simulink model "valid_rst"  (Simulink 9.2)
settings: Solver=ode45  StartTime=0.0  StopTime=1.0  RelTol=1e-3  EnableMultiTasking=on
values from neighbouring files (symbols this model uses):
  Ks = 0.157    [nxt_rst.m]
  R = double(vpa(coeffs(collect(expand(eval(Ax*R0))),z_),Acc))    [nxt_rst.m]
  S = double(vpa(coeffs(collect(expand(eval((1-z_)^p*Bx*S2))),z_),Acc))    [nxt_rst.m]
  T = double(vpa(coeffs(collect(expand(eval(Ax*T0))),z_),Acc))    [nxt_rst.m]
  tau = 0.0667    [nxt_rst.m]
  Te = 0.01    [nxt_rst.m]
settings Model: Creator=Jacques GANGLOFF  LastModifiedBy=jacques
settings OptimizationCC: ExpressionDepthLimit=2147483647  InitFltsAndDblsToZero=on
settings DebuggingCC: SolverPrmCheckMsg=warning

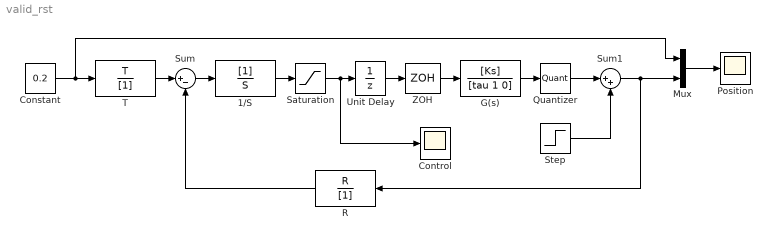
== system valid_rst ==
  1/S : DiscreteFilter  Denominator=S  SampleTime=Te
  Constant : Constant  Value=0.2
  Control : Scope
  G(s) : TransferFcn  Numerator=[Ks]  Denominator=[tau 1 0]
  Mux : Mux  Inputs=2
  Position : Scope
  Quantizer : Quantizer  QuantizationInterval=1/180*pi
  R : DiscreteFilter  Numerator=R  Denominator=[1]  SampleTime=Te
  Saturation : Saturate  UpperLimit=100  LowerLimit=-100
  Step : Step  Time=0.5  After=0.1  SampleTime=0
  Sum : Sum  Inputs=|+-
  Sum1 : Sum  Inputs=|++
  T : DiscreteFilter  Numerator=T  Denominator=[1]  SampleTime=Te
  Unit Delay : UnitDelay  SampleTime=-1
  ZOH : ZeroOrderHold  SampleTime=Te
  wires:
  Constant/1 -> T/1, Mux/1
  T/1 -> Sum/1
  Sum/1 -> 1/S/1
  1/S/1 -> Saturation/1
  ZOH/1 -> G(s)/1
  G(s)/1 -> Quantizer/1
  R/1 -> Sum/2
  Mux/1 -> Position/1
  Quantizer/1 -> Sum1/1
  Sum1/1 -> Mux/2, R/1
  Step/1 -> Sum1/2
  Saturation/1 -> Control/1, Unit Delay/1
  Unit Delay/1 -> ZOH/1
